simulink model "get_flight_data"  (R2021b)
settings: Solver=VariableStepAuto  StartTime=0.0  StopTime=inf  RelTol=1e-3
model workspace (MAT data in the model file):
  enableTransmit = 0
libraries: instrumentlib x4
settings Model: Creator=Vladik  LastModifiedBy=Vladik

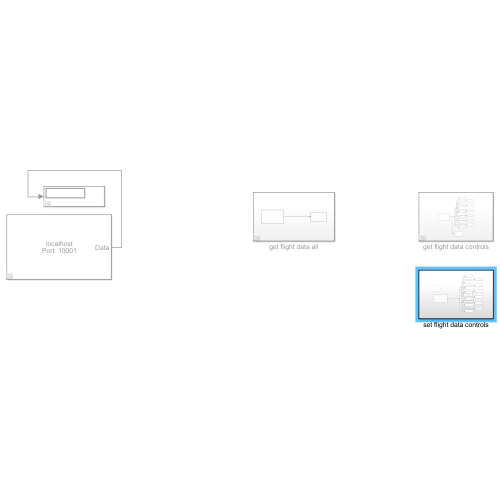
[thumbnail: Simulink's stored preview of the top-level diagram]
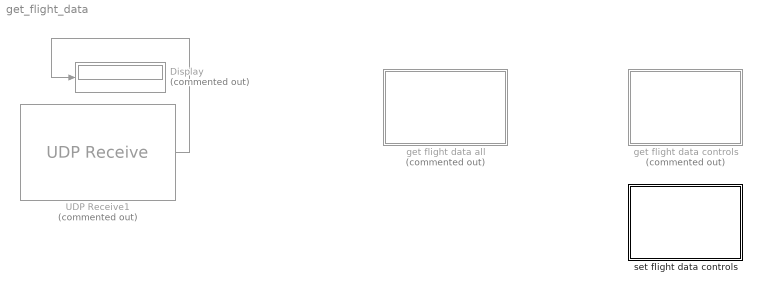
== system get_flight_data ==
  Display : Display  Commented=on
  UDP Receive1 : instrumentlib/UDP Receive  Commented=on  Host=localhost  Port=10001  LocalPort=10001  EnablePortSharing=off  GetLatestData=off  DataSize="[1  1]"  DataType=ASCII  ASCIIFormatting=%f  Terminator=LF  ByteOrder=BigEndian  EnableBlockingMode=on  Timeout=10  SampleTime=0.01  LocalAddress=localhost
  get flight data all : Subsystem  Commented=on
  get flight data controls : Subsystem  Commented=on
  set flight data controls : Subsystem
  wires:
  UDP Receive1/1 -> Display/1

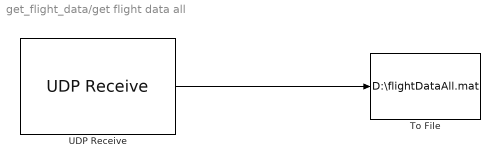
== system get_flight_data/get flight data all ==
  To File : ToFile  Filename=D:\flightDataAll.mat  MatrixName=flight_data_all
  UDP Receive : instrumentlib/UDP Receive  Host=localhost  Port=10000  LocalPort=10000  EnablePortSharing=off  GetLatestData=off  DataSize="[1  35]"  DataType=ASCII  ASCIIFormatting=%f %f %f %f %f %f %f %f %f %f %f %f %f %f %f %f %f %f %f %f %f %f %f %f %f %f %f %f %f %f %f %f %f %f %f  Terminator=LF  ByteOrder=BigEndian  EnableBlockingMode=on  Timeout=10  SampleTime=0.1  LocalAddress=localhost
  wires:
  UDP Receive/1 -> To File/1

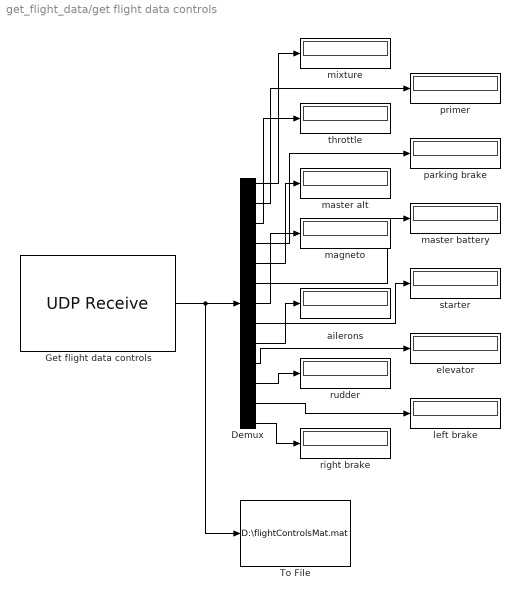
== system get_flight_data/get flight data controls ==
  Demux : Demux  Outputs=13
  Get flight data controls : instrumentlib/UDP Receive  Host=localhost  Port=10000  LocalPort=10000  EnablePortSharing=off  GetLatestData=off  DataSize="[1  13]"  DataType=ASCII  ASCIIFormatting=%f %d %f %d %d %d %d %d %f %f %f %d %d  Terminator=LF  ByteOrder=BigEndian  EnableBlockingMode=on  Timeout=10  SampleTime=0.1  LocalAddress=localhost
  To File : ToFile  Filename=D:\flightControlsMat.mat  MatrixName=flight_controls  SampleTime=0.01
  ailerons : Display
  elevator : Display
  left brake : Display
  magneto : Display
  master alt : Display
  master battery : Display
  mixture : Display
  parking brake : Display
  primer : Display
  right brake : Display
  rudder : Display
  starter : Display
  throttle : Display
  wires:
  Demux/2 -> primer/1
  Demux/1 -> mixture/1
  Demux/3 -> throttle/1
  Demux/6 -> master battery/1
  Demux/8 -> starter/1
  Demux/13 -> right brake/1
  Demux/5 -> master alt/1
  Demux/11 -> rudder/1
  Get flight data controls/1 -> To File/1, Demux/1
  Demux/12 -> left brake/1
  Demux/10 -> elevator/1
  Demux/7 -> magneto/1
  Demux/4 -> parking brake/1
  Demux/9 -> ailerons/1

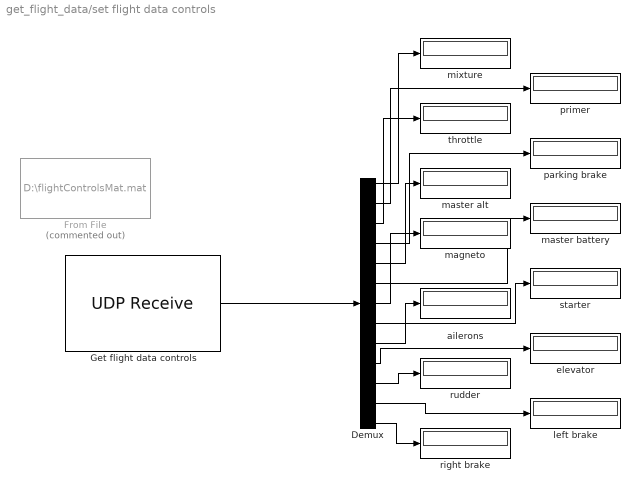
== system get_flight_data/set flight data controls ==
  Demux : Demux  Outputs=13
  From File : FromFile  Commented=on  FileName=D:\flightControlsMat.mat  SampleTime=0.01
  Get flight data controls : instrumentlib/UDP Receive  Host=localhost  Port=10001  LocalPort=10001  EnablePortSharing=off  GetLatestData=off  DataSize="[1  13]"  DataType=ASCII  ASCIIFormatting=%f %d %f %d %d %d %d %d %f %f %f %d %d  Terminator=LF  ByteOrder=BigEndian  EnableBlockingMode=on  Timeout=10  SampleTime=0.1  LocalAddress=localhost
  ailerons : Display
  elevator : Display
  left brake : Display
  magneto : Display
  master alt : Display
  master battery : Display
  mixture : Display
  parking brake : Display
  primer : Display
  right brake : Display
  rudder : Display
  starter : Display
  throttle : Display
  wires:
  Demux/2 -> primer/1
  Demux/1 -> mixture/1
  Demux/3 -> throttle/1
  Demux/6 -> master battery/1
  Demux/8 -> starter/1
  Demux/13 -> right brake/1
  Demux/5 -> master alt/1
  Demux/11 -> rudder/1
  Demux/12 -> left brake/1
  Demux/10 -> elevator/1
  Demux/7 -> magneto/1
  Demux/4 -> parking brake/1
  Demux/9 -> ailerons/1
  Get flight data controls/1 -> Demux/1
